simulink model "counter"  (R2020a)
settings: Solver=VariableStepAuto  StartTime=0.0  StopTime=10.0  RelTol=1e-3
settings Model: Creator=aishw  LastModifiedBy=aishw

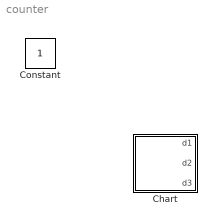
== system counter ==
  Chart : Stateflow chart  TreatAsAtomicUnit=on
  Constant : Constant

== stateflow chart counter/Chart ==
  state digit1 [parallel]
    settings: executionOrder=1
    state one
      en:  d1 = 1;
    state zero
      en: d1 = 0;
    state two
      en: d1 = 2;
    digit1.one -> digit1.two : inputclick
    digit1.zero -> digit1.one : inputclick
    (default) -> digit1.zero
    digit1.two -> digit1.zero : inputclick/{digit2.inc2;}
  state digit2 [parallel]
    settings: executionOrder=2
    state one
      en:  d2 = 1;
    state zero
      en: d2 = 0;
    state two
      en: d2 = 2;
    digit2.one -> digit2.two : inc2
    digit2.zero -> digit2.one : inc2
    (default) -> digit2.zero
    digit2.two -> digit2.zero : inc2/{digit3.inc3;}
  state digit3 [parallel]
    settings: executionOrder=3
    state one
      en:  d3 = 1;
    state zero
      en: d3 = 0;
    state two
      en: d3 = 2;
    digit3.one -> digit3.two : inc3
    digit3.zero -> digit3.one : inc3
    (default) -> digit3.zero
    digit3.two -> digit3.zero : inc3
  data: d1 output; d2 output; d3 output
  events: inputclick local FUNCTION_CALL_EVENT; inc2 local FUNCTION_CALL_EVENT; inc3 local FUNCTION_CALL_EVENT
